simulink model "FAT_F1_F2_temp2(1)"  (R2021b)
settings: Solver=VariableStepAuto  StartTime=0.0  StopTime=5  FixedStep=0.01  RelTol=1e-3
settings Model: Creator=admin  LastModifiedBy=ASUS
settings SolverCC: AlgebraicLoopSolver=TrustRegion
settings DataIOCC: SaveFormat=StructureWithTime
settings OptimizationCC: LifeSpan=inf
settings DebuggingCC: SFExecutionAtInitializationDiag=none  SFMachineParentedDataDiag=warning  ArithmeticOperatorsInVariantConditions=warning
settings HardwareCC: ProdBitPerSizeT=32  ProdBitPerPtrDiffT=32  ProdWordSize=32  ProdHWDeviceType=Specified
settings SFSimCC: CustomCodeUndefinedFunction=UseInterfaceOnly
settings CodeAppCC: StateflowObjectComments=on

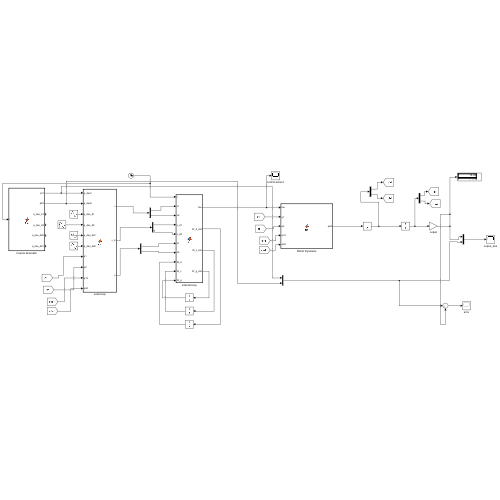
[thumbnail: Simulink's stored preview of the top-level diagram]
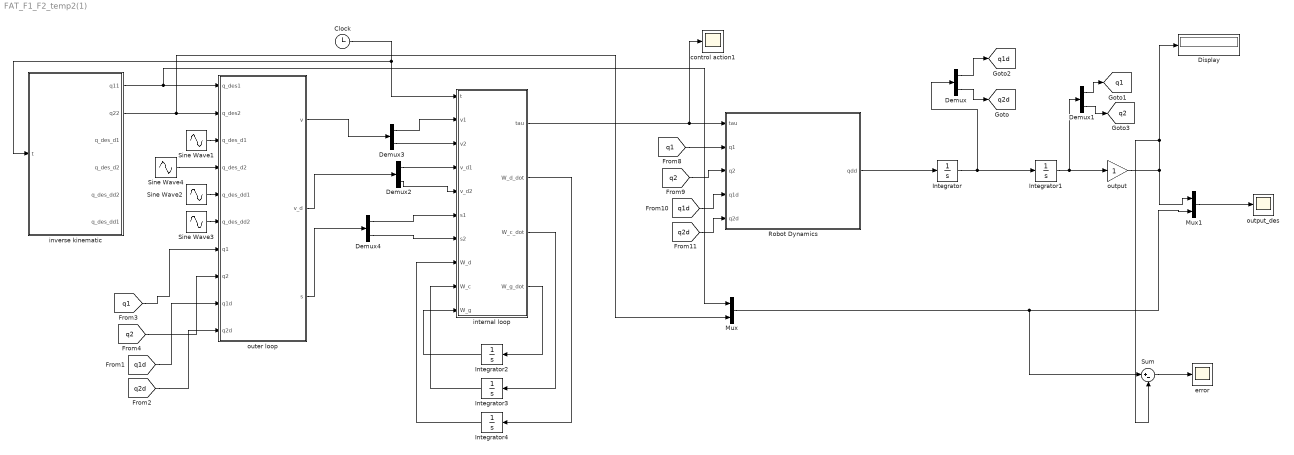
== system FAT_F1_F2_temp2(1) ==
  Clock : Clock
  Demux{,1..4} (5 alike) : Demux  Outputs=2
  Display : Display
  Integrator : Integrator  InitialCondition=[0;0]
  Integrator1 : Integrator  InitialCondition=[0;0]
  Integrator2 : Integrator  InitialCondition=rand(3,2)
  Integrator3 : Integrator  InitialCondition=rand(6,2)
  Integrator4 : Integrator  InitialCondition=rand(6,2)
  Mux : Mux  Inputs=2
  Mux1 : Mux  Inputs=2
  Robot Dynamics : MATLAB Function  TreatAsAtomicUnit=on
  Sine Wave{1..4} (4 alike) : Sin  SampleTime=0
  Sum : Sum  Inputs=|+-
  control action1 : Scope
  error : Scope
  internal loop : MATLAB Function  TreatAsAtomicUnit=on
  inverse kinematic : MATLAB Function  TreatAsAtomicUnit=on
  outer loop : MATLAB Function  TreatAsAtomicUnit=on
  output : Gain
  output_des : Scope
  tag scope: q1=global, q1d=global, q2=global, q2d=global
  wires:
  [q2] -> Robot Dynamics/3(q2)
  [q1d] -> Robot Dynamics/4(q1d)
  [q1] -> Robot Dynamics/2(q1)
  [q2d] -> Robot Dynamics/5(q2d)
  Integrator/1 -> Demux/1, Integrator1/1
  output/1 -> Sum/2, Display/1, Mux1/1
  Demux1/1 -> [q1]
  Integrator1/1 -> Demux1/1, output/1
  Robot Dynamics/1(qdd) -> Integrator/1
  Demux/2 -> [q2d]
  Demux1/2 -> [q2]
  Demux/1 -> [q1d]
  internal loop/1(tau) -> control action1/1, Robot Dynamics/1(tau)
  internal loop/4(W_g_dot) -> Integrator2/1
  internal loop/3(W_c_dot) -> Integrator3/1
  internal loop/2(W_d_dot) -> Integrator4/1
  Integrator4/1 -> internal loop/8(W_d)
  Integrator3/1 -> internal loop/9(W_c)
  Integrator2/1 -> internal loop/10(W_g)
  [q1] -> outer loop/7(q1)
  [q2] -> outer loop/8(q2)
  [q1d] -> outer loop/9(q1d)
  [q2d] -> outer loop/10(q2d)
  Clock/1 -> inverse kinematic/1(t), internal loop/1(t)
  outer loop/2(v_d) -> Demux2/1
  Demux2/1 -> internal loop/4(v_d1)
  Demux2/2 -> internal loop/5(v_d2)
  outer loop/1(v) -> Demux3/1
  Demux3/1 -> internal loop/2(v1)
  Demux3/2 -> internal loop/3(v2)
  outer loop/3(s) -> Demux4/1
  Demux4/1 -> internal loop/6(s1)
  Demux4/2 -> internal loop/7(s2)
  Mux/1 -> Sum/1, Mux1/2
  Mux1/1 -> output_des/1
  Sum/1 -> error/1
  inverse kinematic/2(q22) -> Mux/2, outer loop/2(q_des2)
  inverse kinematic/1(q11) -> Mux/1, outer loop/1(q_des1)
  Sine Wave3/1 -> outer loop/6(q_des_dd2)
  Sine Wave2/1 -> outer loop/5(q_des_dd1)
  Sine Wave1/1 -> outer loop/3(q_des_d1)
  Sine Wave4/1 -> outer loop/4(q_des_d2)

== matlab function FAT_F1_F2_temp2(1)/Robot Dynamics ==
  data: tau input; q1 input; qdd output; q2 input; q1d input; q2d input
function qdd = fcn(tau,q1,q2,q1d,q2d)

% q1=q(1);
% q2=q(2);
% 
% q1d=qd(1);
% q2d=qd(2);

qd = [q1d;q2d];

m1=.1;
m2=.1;

I1=.01;
I2=.01;

l1=.12;
l2=.1;

lc1=l1/2;
lc2=l2/2;


g=9.8;



d11=m1*lc1^2+m2*(l1^2+lc2^2+2*l1*lc2^2+2*l1*l2*cos(q2))+I1+I2;
d12=m2*(lc2^2+l1*l2*cos(q2))+I2;
d22=m2*lc2^2+I2;

h=-m2*l1*lc2*sin(q2);

c121=h;
c211=h;
c112=-h;
c221=h;



M=[d11,d12;d12,d22];
C=[c121*q2d,c211*q1d+c221*q2d;c112*q1d,0];
G=[(m1*lc1+m2*l1)*g*cos(q1)+m2*lc2*g*cos(q1+q2);m2*lc2*cos(q1+q2)];


qdd=pinv(M)*((tau)-C*qd-G);

== matlab function FAT_F1_F2_temp2(1)/internal loop ==
  data: t input; tau output; v1 input; v2 input; v_d1 input; v_d2 input; s1 input; s2 input; W_d input; W_c input; W_g input; W_d_dot output; W_c_dot output; W_g_dot output
function [tau,W_d_dot,W_c_dot,W_g_dot] = fcn(t,v1,v2,v_d1,v_d2,s1,s2,W_d,W_c,W_g)
s = [s1;s2];
v = [v1;v2];
v_d = [v_d1;v_d2];
fn = 5;
%sinwt w =50
zz = [1;sin(fn*t);sin(2*fn*t)];

Zd = [zz,zeros(3,1);zeros(3,1),zz];

Zc = Zd;
Zg = zz;

D_hat = W_d'*Zd;
C_hat = W_c'*Zc;
g_hat = W_g'*Zg;

Qd = 100*eye(6);
Qc = 100*eye(6);
Qg = 100*eye(3);

Kd = [10 0;0 10];
robust = [sign(s(1,1));sign(s(2,1))];
tau = g_hat+D_hat*v_d+C_hat*v-Kd*s-0.001*robust;
W_d_dot= -pinv(Qd)*Zd*s*v_d';
W_c_dot= -pinv(Qc)*Zc*s*v';
W_g_dot= -pinv(Qg)*Zg*s';

== matlab function FAT_F1_F2_temp2(1)/outer loop ==
  data: q_des1 input; v output; q_des2 input; q_des_d1 input; q_des_d2 input; q_des_dd1 input; q_des_dd2 input; q1 input; q2 input; q1d input; q2d input; v_d output; s output
function [v,v_d,s] = fcn(q_des1,q_des2,q_des_d1,q_des_d2,q_des_dd1,q_des_dd2,q1,q2,q1d,q2d)
gamma = 10;
q_des = [q_des1;q_des2];
q_des_d = [q_des_d1;q_des_d2];
q_des_dd = [q_des_dd1;q_des_dd2];
q = [q1;q2];
qd = [q1d;q2d];

e = q-q_des;
e_d = qd-q_des_d;

s = e_d+gamma*e;
v = q_des_d-gamma*e;
v_d = q_des_dd-gamma*e_d;

== matlab function FAT_F1_F2_temp2(1)/inverse kinematic ==
  data: q11 output; q22 output; t input; q_des_d1 output; q_des_d2 output; q_des_dd2 output; q_des_dd1 output
% function [q1,q12, q21,q2,q_des_d1,q_des_d2,q_des_dd1,q_des_dd2] = fcn(Xee,Yee,t)
% % DH parameters
% l1=.15;
% l2=.15;
% % d1=d2=0
% %temp1 = 2*l1*l2;
% %temp2 = Xee^2+Yee^2-l1^2-l2^2;
% %temp = temp2/temp1
% %q2 = acos((temp2/temp1));
% 
% %k = (l1^2-l2^2+Xee^2+Yee^2)/(2*l1);
% %alfa = [k*Yee - Xee*sqrt(Xee^2+Yee^2-k^2)]/(Xee^2+Yee^2);
% %q11 = asin(alfa);
% %alfa2 = [k*Yee + Xee*sqrt(Xee^2+Yee^2-k^2)]/(Xee^2+Yee^2);
% %q12 = asin(alfa2);
% Xee_d   = ((cos(t))*(exp(cos(t))-2*cos(4*t)+((sin(1/12*t))^5)))+(((sin(t))*exp((cos(t)))- 8*sin(4*t)+5*(sin(1/12*t)^4)*1/12*cos(1/12*t))*(sin(t)));
% Xee_dd  = diff(Xee_d);
% Yee_d   = ((sin(t))*(exp(cos(t))-2*cos(4*t)+((sin(1/12*t))^5)))+(((sin(t))*exp((cos(t)))- 8*sin(4*t)+5*(sin(1/12*t)^4)*1/12*cos(1/12*t))*(cos(t)));
% Yee_dd  = diff(Yee_d);
% 
% D = (Xee^2+Yee^2-l1^2-l2^2)/(2*l1*l2);
% D_d = ((2*Xee*Xee_d+2*Yee*Yee_d)*(2*l1*l2))/((2*l1*l2)^2);
% D_dd = ((2*(Xee_d)^2+2*Xee_dd*Xee+(2*(Yee_d)^2+2*Yee_dd*Yee)*(2*l1*l2)^2))/((2*l1*l2)^4);
% 
% q22 = atan2(sqrt(1-D^2),D);
% q21 = atan2(-sqrt(1-D^2),D);
% q22 = atan2(sin(q22),cos(q22));
% if q22<(pi/2)
%     q2=q22;
% else
%     q2=q21;
% end
% %q21 = 0;
% q11 = atan2(Yee,Xee)-atan2(l2*sin(q22),(l1+l2*cos(q22)));
% q12 = atan2(Yee,Xee)-atan2(l2*sin(q21),(l1+l2*cos(q21)));
% q11 = atan2(sin(q11),cos(q11));
% q12 = atan2(sin(q12),cos(q12));
% % if q11<(pi/2)
% %     q1=q11;
% % else
% %     q1=q12;
% % end
% q_des_d1 =(Yee_d*Xee-Xee_d*Yee)/(Xee^2+Yee^2) -(((l2*cos(q22)*(l1+l2*cos(q22)))+((l2*sin(q22))^2))/(((l2*sin(q22))^2)+((l1+l2*cos(q22)))^2));
% 
% q_des_d2 = (0.5*1/((1-D^2)^2))*-2*D_d*(D^2)-D_d*sqrt(1-D^2);
% q_des_dd2 = ((-D*D_d+2*D*D_d)*((1-D^2)^2+D^2)-(-2*D*D_d-2*(D_dd*D+D_d^2)))/(((1-D^2)^2+D^2)^2);
% %q12 = 0;
% q_des_dd1 = ((Yee_dd*Xee)*(Xee^2+Yee^2)-(2*Xee*Xee_d+2*Yee*Yee_d)*( Yee_d*Xee-Xee_d*Yee))/((Xee^1+Yee^2)^2)-(((-l2*l1*sin(q22)-l2^2*sin(q22)-l2^2*sin(q22)+2*l1*sin(q22)*cos(q22))*((l2*sin(q22))^2)+((l1+l2*cos(q22)))^2)-(2*l1*sin(q22)*cos(q22)-2*l2*cos(q22)*sin(q22)-2*l1*l2*sin(q22))*(((l2*cos(q22)*(l1+l2*cos(q22)))+((l2*sin(q22))^2))))/(((((l2*sin(q22))^2)+((l1+l2*cos(q22)))^2))^2);
% end



%%%%%%%%%%%%%%%%%%%%%%%%%%%%%%%%%%%%%%%%%%%%%%%%%%%%%%%%%%
% function [q11,q22,q_des_d1,q_des_d2,q_des_dd1,q_des_dd2,dm,D,temp1,temp2,temp3,test,test1]  = fcn(t)
 
%DH parameters
% l1=.15;
% l2=.15;
% % d1=d2=0
% %temp1 = 2*l1*l2;
% %temp2 = Xee^2+Yee^2-l1^2-l2^2;
% %temp = temp2/temp1
% %q2 = acos((temp2/temp1));
% 
% %k = (l1^2-l2^2+Xee^2+Yee^2)/(2*l1);
% %alfa = [k*Yee - Xee*sqrt(Xee^2+Yee^2-k^2)]/(Xee^2+Yee^2);
% %q11 = asin(alfa);
% %alfa2 = [k*Yee + Xee*sqrt(Xee^2+Yee^2-k^2)]/(Xee^2+Yee^2);
% %q12 = asin(alfa2);
% Xee = (sin(t))*(exp(cos(t))-2*cos(4*t)+((sin(1/12*t))^5));
% Yee =(cos(t))*(exp(cos(t))-2*cos(4*t)+((sin(1/12*t))^5));
% Xee_d=sin(t)*(8*sin(4*t) + (5*cos(t/12)*sin(t/12)^4)/12 - exp(cos(t))*sin(t)) + cos(t)*(exp(cos(t)) - 2*cos(4*t) + sin(t/12)^5);
% Yee_d=cos(t)*(8*sin(4*t) + (5*cos(t/12)*sin(t/12)^4)/12 - exp(cos(t))*sin(t)) - sin(t)*(exp(cos(t)) - 2*cos(4*t) + sin(t/12)^5);
% Xee_dd=sin(t)*(32*cos(4*t) - exp(cos(t))*cos(t) + (5*cos(t/12)^2*sin(t/12)^3)/36 - (5*sin(t/12)^5)/144 + exp(cos(t))*sin(t)^2) - sin(t)*(exp(cos(t)) - 2*cos(4*t) + sin(t/12)^5) + 2*cos(t)*(8*sin(4*t) + (5*cos(t/12)*sin(t/12)^4)/12 - exp(cos(t))*sin(t));
% Yee_dd=cos(t)*(32*cos(4*t) - exp(cos(t))*cos(t) + (5*cos(t/12)^2*sin(t/12)^3)/36 - (5*sin(t/12)^5)/144 + exp(cos(t))*sin(t)^2) - cos(t)*(exp(cos(t)) - 2*cos(4*t) + sin(t/12)^5) - 2*sin(t)*(8*sin(4*t) + (5*cos(t/12)*sin(t/12)^4)/12 - exp(cos(t))*sin(t));
% 
% % Xee = 16*(sin(t)^3);
% % Yee = 13*cos(t)-5*cos(2*t)-2*cos(3*t)-cos(4*t);
% % Xee_d = 16*3*(sin(t)^2)*cos(t);
% % Yee_d =10*sin(2*t) + 6*sin(3*t) + 4*sin(4*t) - 13*sin(t);
% % Xee_dd=96*cos(t)^2*sin(t) - 48*sin(t)^3;
% % Yee_dd=20*cos(2*t) + 18*cos(3*t) + 16*cos(4*t) - 13*cos(t);
% 
% D = (Xee^2+Yee^2-l1^2-l2^2)/(2*l1*l2);
% D_d = ((2*Xee*Xee_d+2*Yee*Yee_d)*(2*l1*l2))/((2*l1*l2)^2);
% D_dd = ((2*(Xee_d)^2+2*Xee_dd*Xee+(2*(Yee_d)^2+2*Yee_dd*Yee)*(2*l1*l2)^2))/((2*l1*l2)^4);
% % 
% % l1=.15;
% % l2=.15;
% % Xee = (sin(t))*(exp(cos(t))-2*cos(4*t)+((sin(1/12*t))^5));
% % Yee =(cos(t))*(exp(cos(t))-2*cos(4*t)+((sin(1/12*t))^5));
% % Xee_d   = ((cos(t))*(exp(cos(t))-2*cos(4*t)+((sin(1/12*t))^5)))+(((sin(t))*exp((cos(t)))- 8*sin(4*t)+5*(sin(1/12*t)^4)*1/12*cos(1/12*t))*(sin(t)));
% % 
% % Yee_d   = ((sin(t))*(exp(cos(t))-2*cos(4*t)+((sin(1/12*t))^5)))+(((sin(t))*exp((cos(t)))- 8*sin(4*t)+5*(sin(1/12*t)^4)*1/12*cos(1/12*t))*(cos(t)));
% 
% % q_des_d1=(Yee_d*Xee-Xee_d*Yee)/(Xee^2+Yee^2);
% % D = (Xee^2+Yee^2-l1^2-l2^2)/(2*l1*l2);
% dm=sqrt(abs(1-D^2));
% temp=dm/D;
% test=sin(temp)/cos(temp);
% q22=atan(test);
% if (1-D^2)<0
%     q22 =  atan2(-dm,D);
% else 
%     q22 = atan2(dm,D);
% end
% q22 = atan2(sqrt(1-D^2),D);
%%%%%%%%%%%%%%%%%%%%%%%%%%%%%%%%%%%%%%%%%%%%%%%%%%%%%%%
% l1=1.5;
% l2=1.5;
% % d1=d2=0
% %temp1 = 2*l1*l2;
% %temp2 = Xee^2+Yee^2-l1^2-l2^2;
% %temp = temp2/temp1
% %q2 = acos((temp2/temp1));
% 
% %k = (l1^2-l2^2+Xee^2+Yee^2)/(2*l1);
% %alfa = [k*Yee - Xee*sqrt(Xee^2+Yee^2-k^2)]/(Xee^2+Yee^2);
% %q11 = asin(alfa);
% %alfa2 = [k*Yee + Xee*sqrt(Xee^2+Yee^2-k^2)]/(Xee^2+Yee^2);
% %q12 = asin(alfa2);
% % Xee = (sin(t))*(exp(cos(t))-2*cos(4*t)+((sin(1/12*t))^5));
% % Yee =(cos(t))*(exp(cos(t))-2*cos(4*t)+((sin(1/12*t))^5));
% % Xee_d=sin(t)*(8*sin(4*t) + (5*cos(t/12)*sin(t/12)^4)/12 - exp(cos(t))*sin(t)) + cos(t)*(exp(cos(t)) - 2*cos(4*t) + sin(t/12)^5);
% % Yee_d=cos(t)*(8*sin(4*t) + (5*cos(t/12)*sin(t/12)^4)/12 - exp(cos(t))*sin(t)) - sin(t)*(exp(cos(t)) - 2*cos(4*t) + sin(t/12)^5);
% % Xee_dd=sin(t)*(32*cos(4*t) - exp(cos(t))*cos(t) + (5*cos(t/12)^2*sin(t/12)^3)/36 - (5*sin(t/12)^5)/144 + exp(cos(t))*sin(t)^2) - sin(t)*(exp(cos(t)) - 2*cos(4*t) + sin(t/12)^5) + 2*cos(t)*(8*sin(4*t) + (5*cos(t/12)*sin(t/12)^4)/12 - exp(cos(t))*sin(t));
% % Yee_dd=cos(t)*(32*cos(4*t) - exp(cos(t))*cos(t) + (5*cos(t/12)^2*sin(t/12)^3)/36 - (5*sin(t/12)^5)/144 + exp(cos(t))*sin(t)^2) - cos(t)*(exp(cos(t)) - 2*cos(4*t) + sin(t/12)^5) - 2*sin(t)*(8*sin(4*t) + (5*cos(t/12)*sin(t/12)^4)/12 - exp(cos(t))*sin(t));
% 
% Xee = 16*(sin(t)^3);
% Yee = 13*cos(t)-5*cos(2*t)-2*cos(3*t)-cos(4*t);
% Xee_d = 16*3*(sin(t)^2)*cos(t);
% Yee_d =10*sin(2*t) + 6*sin(3*t) + 4*sin(4*t) - 13*sin(t);
% Xee_dd=96*cos(t)^2*sin(t) - 48*sin(t)^3;
% Yee_dd=20*cos(2*t) + 18*cos(3*t) + 16*cos(4*t) - 13*cos(t);
% 
% D = (Xee^2+Yee^2-l1^2-l2^2)/(2*l1*l2);
% D_d = ((2*Xee*Xee_d+2*Yee*Yee_d)*(2*l1*l2))/((2*l1*l2)^2);
% D_dd = ((2*(Xee_d)^2+2*Xee_dd*Xee+(2*(Yee_d)^2+2*Yee_dd*Yee)*(2*l1*l2)^2))/((2*l1*l2)^4);
% % 
% % l1=.15;
% % l2=.15;
% % Xee = (sin(t))*(exp(cos(t))-2*cos(4*t)+((sin(1/12*t))^5));
% % Yee =(cos(t))*(exp(cos(t))-2*cos(4*t)+((sin(1/12*t))^5));
% % Xee_d   = ((cos(t))*(exp(cos(t))-2*cos(4*t)+((sin(1/12*t))^5)))+(((sin(t))*exp((cos(t)))- 8*sin(4*t)+5*(sin(1/12*t)^4)*1/12*cos(1/12*t))*(sin(t)));
% % 
% % Yee_d   = ((sin(t))*(exp(cos(t))-2*cos(4*t)+((sin(1/12*t))^5)))+(((sin(t))*exp((cos(t)))- 8*sin(4*t)+5*(sin(1/12*t)^4)*1/12*cos(1/12*t))*(cos(t)));
% 
% % q_des_d1=(Yee_d*Xee-Xee_d*Yee)/(Xee^2+Yee^2);
% % D = (Xee^2+Yee^2-l1^2-l2^2)/(2*l1*l2);
% temp1=(1-D^2);
% temp2=(temp1);
% dm=sqrt(abs(1-D^2));
% temp3=dm/D;
% test=sin(temp3)/cos(temp3);
% test1=atan(test);
% q22=atan(test);
% 
% 
% 
% 
% 
% 
% 
% % q21 = 0
% % % q22 = atan2(sin(q22),cos(q22));
% % %q21 = 0;
%  q11 = atan2(Yee,Xee)-atan2(l2*sin(q22),(l1+l2*cos(q22)));
% % q12 = atan2(Yee,Xee)-atan2(l2*sin(q22),(l1+l2*cos(q21)));
%  q11 = atan2(sin(q11),cos(q11));
% % % q12 = atan2(sin(q12),cos(q12));
%  q_des_d1 =(Yee_d*Xee-Xee_d*Yee)/(Xee^2+Yee^2) -(((l2*cos(q22)*(l1+l2*cos(q22)))+((l2*sin(q22))^2))/(((l2*sin(q22))^2)+((l1+l2*cos(q22)))^2));
% % % 
% %  q_des_d2 = (0.5*1/((1-D^2)^2))*-2*D_d*(D^2)-D_d*sqrt(1-D^2);
% dm_d = diff(sqrt(abs(1-D^2)));
% temp_d = (dm_d*D-D_d*dm)/D^2;
% % q_des_d2= ((temp_d*cos(temp)*cos(temp))-(temp_d*-sin(temp)*sin(temp)))/ (cos(temp)^2);
% q_des_d2=(0.5*1/((1-D^2)^2))*-2*D_d*(D^2)-D_d*sqrt(abs(1-D^2));
%  q_des_dd2 = ((-D*D_d+2*D*D_d)*((1-D^2)^2+D^2)-(-2*D*D_d-2*(D_dd*D+D_d^2)))/(((1-D^2)^2+D^2)^2);
% 
% % % %q12 = 0;
%  q_des_dd1 = ((Yee_dd*Xee)*(Xee^2+Yee^2)-(2*Xee*Xee_d+2*Yee*Yee_d)*( Yee_d*Xee-Xee_d*Yee))/((Xee^1+Yee^2)^2)-(((-l2*l1*sin(q22)-l2^2*sin(q22)-l2^2*sin(q22)+2*l1*sin(q22)*cos(q22))*((l2*sin(q22))^2)+((l1+l2*cos(q22)))^2)-(2*l1*sin(q22)*cos(q22)-2*l2*cos(q22)*sin(q22)-2*l1*l2*sin(q22))*(((l2*cos(q22)*(l1+l2*cos(q22)))+((l2*sin(q22))^2))))/(((((l2*sin(q22))^2)+((l1+l2*cos(q22)))^2))^2);
% % % q_des_d1 = diff(sin(t));
% % % q_des_d2= diff(q11);
% % q_des_dd1=diff(q_des_d1);
% % q_des_dd2 = diff(q_des_d2);
%%%%%%%%%%%%%%%%%%%%%%%%%%%%%%%%%%%%%%%%%%%%%%%%%%%%%%%%%%%%%%%%%%%%%%%%%%%%%%%%%%%%%%%%%%%%%%%%%%%%%%
%with diff matlab
%%ghalb dorost vali derivative hamchenan 0 q22 ro 0 mide
% function [q11,q22,q_des_d1,q_des_d2,q_des_dd1,q_des_dd2,temp1]  = fcn(t)
% l1=1.5;
% l2=1.5;
% T=t
% Xee = 16*(sin(t)^3);
% Yee = 13*cos(t)-5*cos(2*t)-2*cos(3*t)-cos(4*t);
% Xee_d = 16*3*(sin(t)^2)*cos(t);
% Yee_d =10*sin(2*t) + 6*sin(3*t) + 4*sin(4*t) - 13*sin(t);
% Xee_dd=96*cos(t)^2*sin(t) - 48*sin(t)^3;
% Yee_dd=20*cos(2*t) + 18*cos(3*t) + 16*cos(4*t) - 13*cos(t);
% D = (0.001*Xee^2+0.001*Yee^2-l1^2-l2^2)/(2*l1*l2);
% D_d=(4*sin(t)*(423*cos(t) + 210*cos(t)^2 - 808*cos(t)^3 + 680*cos(t)^4 + 480*cos(t)^5 - 448*cos(t)^6 - 256*cos(t)^7 - 76))/9;
% D_dd=(4360*cos(t)^2)/3 - (1984*cos(t))/9 - (8360*cos(t)^3)/9 - (22528*cos(t)^4)/9 + (24352*cos(t)^5)/9 + (18688*cos(t)^6)/9 - (12544*cos(t)^7)/9 - (8192*cos(t)^8)/9 - 188;
% q22 = atan2((1-D^2),D);
% temp1=(1-D^2);
% for T=1:4.5
%  q11 = 0;
% end 
% for T=4.5:10
% 
%     q11 = atan2(Yee,Xee)-atan2(l2*sin(q22),(l1+l2*cos(q22)))+pi/2;
% end
%  q_des_d1 =(Yee_d*Xee-Xee_d*Yee)/(Xee^2+Yee^2) -(((l2*cos(q22)*(l1+l2*cos(q22)))+((l2*sin(q22))^2))/(((l2*sin(q22))^2)+((l1+l2*cos(q22)))^2));
% q_des_d2=(0.5*1/((1-D^2)^2))*-2*D_d*(D^2)-D_d*sqrt(abs(1-D^2));
%  q_des_dd2 = ((-D*D_d+2*D*D_d)*((1-D^2)^2+D^2)-(-2*D*D_d-2*(D_dd*D+D_d^2)))/(((1-D^2)^2+D^2)^2);
% 
% % % %q12 = 0;
%  q_des_dd1 = ((Yee_dd*Xee)*(Xee^2+Yee^2)-(2*Xee*Xee_d+2*Yee*Yee_d)*( Yee_d*Xee-Xee_d*Yee))/((Xee^1+Yee^2)^2)-(((-l2*l1*sin(q22)-l2^2*sin(q22)-l2^2*sin(q22)+2*l1*sin(q22)*cos(q22))*((l2*sin(q22))^2)+((l1+l2*cos(q22)))^2)-(2*l1*sin(q22)*cos(q22)-2*l2*cos(q22)*sin(q22)-2*l1*l2*sin(q22))*(((l2*cos(q22)*(l1+l2*cos(q22)))+((l2*sin(q22))^2))))/(((((l2*sin(q22))^2)+((l1+l2*cos(q22)))^2))^2);
% % % q_des_d1 = diff(sin(t));
%%%%%%%%%%%%%%%%%%%%%%%%%%%%%%%%%%%%%%%%%%%%%%%%%%%%%%%%%%%%%%%%%
%with if
% function [q11,q22,q_des_d1,q_des_d2,q_des_dd1,q_des_dd2,temp1]  = fcn(t,t1)
% l1=1.5;
% l2=1.5;
% T=t
% Xee = 16*(sin(t)^3);
% Yee = 13*cos(t)-5*cos(2*t)-2*cos(3*t)-cos(4*t);
% Xee_d = 16*3*(sin(t)^2)*cos(t);
% Yee_d =10*sin(2*t) + 6*sin(3*t) + 4*sin(4*t) - 13*sin(t);
% Xee_dd=96*cos(t)^2*sin(t) - 48*sin(t)^3;
% Yee_dd=20*cos(2*t) + 18*cos(3*t) + 16*cos(4*t) - 13*cos(t);
% D = (0.001*Xee^2+0.001*Yee^2-l1^2-l2^2)/(2*l1*l2);
% D_d=(4*sin(t)*(423*cos(t) + 210*cos(t)^2 - 808*cos(t)^3 + 680*cos(t)^4 + 480*cos(t)^5 - 448*cos(t)^6 - 256*cos(t)^7 - 76))/9;
% D_dd=(4360*cos(t)^2)/3 - (1984*cos(t))/9 - (8360*cos(t)^3)/9 - (22528*cos(t)^4)/9 + (24352*cos(t)^5)/9 + (18688*cos(t)^6)/9 - (12544*cos(t)^7)/9 - (8192*cos(t)^8)/9 - 188;
% q22 = atan2((1-D^2),D);
% temp1=(1-D^2);
% temp3=atan2(Yee,Xee);
% temp4=-atan2(l2*sin(q22),(l1+l2*cos(q22)));
% if (temp3<-1.5681)
%     temp3=temp3+3;
%     temp4=temp4+3;
%     q11 = temp3+temp4;
% else 
%     q11 = temp3+temp4;
% end
% 
% q11 = atan2(sin(q11),cos(q11));
% 
% to=q11

% 
% % % %q12 = 0;
%  q_des_dd1 = ((Yee_dd*Xee)*(Xee^2+Yee^2)-(2*Xee*Xee_d+2*Yee*Yee_d)*( Yee_d*Xee-Xee_d*Yee))/((Xee^1+Yee^2)^2)-(((-l2*l1*sin(q22)-l2^2*sin(q22)-l2^2*sin(q22)+2*l1*sin(q22)*cos(q22))*((l2*sin(q22))^2)+((l1+l2*cos(q22)))^2)-(2*l1*sin(q22)*cos(q22)-2*l2*cos(q22)*sin(q22)-2*l1*l2*sin(q22))*(((l2*cos(q22)*(l1+l2*cos(q22)))+((l2*sin(q22))^2))))/(((((l2*sin(q22))^2)+((l1+l2*cos(q22)))^2))^2);
% % % q_des_d1 = diff(sin(t));
%%%%%%%%%%%%%%%%%%%%%%%%%%%%%%%%%%%%%%%%%%%%%%%%%%%%%%%%%%%%%%%%%%%%%%%%%%%%%%%%%%%%%55
%if masir barax
 function [q11,q22,q_des_d1,q_des_d2, q_des_dd2,q_des_dd1]= fcn(t)
    l1=1.5;
l2=1.5;
Xee = 16*(sin(t)^3);
Yee = 13*cos(t)-5*cos(2*t)-2*cos(3*t)-cos(4*t);
Xee_d = 16*3*(sin(t)^2)*cos(t);
Yee_d =10*sin(2*t) + 6*sin(3*t) + 4*sin(4*t) - 13*sin(t);
Xee_dd=96*cos(t)^2*sin(t) - 48*sin(t)^3;
Yee_dd=20*cos(2*t) + 18*cos(3*t) + 16*cos(4*t) - 13*cos(t);
D = (0.001*Xee^2+0.001*Yee^2-l1^2-l2^2)/(2*l1*l2);
D_d=(4*sin(t)*(423*cos(t) + 210*cos(t)^2 - 808*cos(t)^3 + 680*cos(t)^4 + 480*cos(t)^5 - 448*cos(t)^6 - 256*cos(t)^7 - 76))/9;
D_dd=(4360*cos(t)^2)/3 - (1984*cos(t))/9 - (8360*cos(t)^3)/9 - (22528*cos(t)^4)/9 + (24352*cos(t)^5)/9 + (18688*cos(t)^6)/9 - (12544*cos(t)^7)/9 - (8192*cos(t)^8)/9 - 188;

% q22 = atan2((1-D^2),D);
temp1=(1-D^2);
temp2=atan2(temp1,1000*D);
q22 = atan2(sqrt(1-D^2),D);
t1=t-5;

    
temp3=atan2(Yee,Xee);
temp4=-atan2(l2*sin(q22),(l1+l2*cos(q22)));
q11 = temp3+temp4;
if (Xee<0)
    Xee = 16*(sin(t1)^3);
Yee = 13*cos(t1)-5*cos(2*t1)-2*cos(3*t1)-cos(4*t1);
Xee_d = 16*3*(sin(t1)^2)*cos(t1);
Yee_d =10*sin(2*t1) + 6*sin(3*t1) + 4*sin(4*t1) - 13*sin(t1);
Xee_dd=96*cos(t1)^2*sin(t1) - 48*sin(t1)^3;
Yee_dd=20*cos(2*t1) + 18*cos(3*t1) + 16*cos(4*t1) - 13*cos(t1);
D = (0.001*Xee^2+0.001*Yee^2-l1^2-l2^2)/(2*l1*l2);
D_d=(4*sin(t1)*(423*cos(t1) + 210*cos(t1)^2 - 808*cos(t1)^3 + 680*cos(t1)^4 + 480*cos(t1)^5 - 448*cos(t1)^6 - 256*cos(t1)^7 - 76))/9;
D_dd=(4360*cos(t1)^2)/3 - (1984*cos(t1))/9 - (8360*cos(t1)^3)/9 - (22528*cos(t1)^4)/9 + (24352*cos(t1)^5)/9 + (18688*cos(t1)^6)/9 - (12544*cos(t1)^7)/9 - (8192*cos(t1)^8)/9 - 188;
temp1=(1-D^2);
temp2=atan2(temp1,1000*D);
q22 = atan2(sqrt(1-D^2),D);
temp3=atan2(Yee,Xee);
temp4=-atan2(l2*sin(q22),(l1+l2*cos(q22)));
q11 = temp3+pi+temp4+pi;
end
q_des_d1 =(Yee_d*Xee-Xee_d*Yee)/(Xee^2+Yee^2) -(((l2*cos(q22)*(l1+l2*cos(q22)))+((l2*sin(q22))^2))/(((l2*sin(q22))^2)+((l1+l2*cos(q22)))^2));
q_des_d2=(0.5*1/((1-D^2)^2))*-2*D_d*(D^2)-D_d*sqrt(abs(1-D^2));
q_des_dd2 = ((-D*D_d+2*D*D_d)*((1-D^2)^2+D^2)-(-2*D*D_d-2*(D_dd*D+D_d^2)))/(((1-D^2)^2+D^2)^2);
q_des_dd1 = (((Yee_dd*Xee)-(Xee_dd*Yee))*(Xee^2+Yee^2)-(2*Xee*Xee_d+2*Yee*Yee_d)*( Yee_d*Xee-Xee_d*Yee))/((Xee^2+Yee^2)^2)-(((-l2*l1*sin(q22)-l2^2*sin(q22)-l2^2*sin(q22)+2*l1*sin(q22)*cos(q22))*((l2*sin(q22))^2)+((l1+l2*cos(q22)))^2)-(2*l1*sin(q22)*cos(q22)-2*l2*cos(q22)*sin(q22)-2*l1*l2*sin(q22))*(((l2*cos(q22)*(l1+l2*cos(q22)))+((l2*sin(q22))^2))))/(((((l2*sin(q22))^2)+((l1+l2*cos(q22)))^2))^2);
